simulink model "IRSensor"  (R2023b)
settings: Solver=FixedStepDiscrete  StartTime=0.0  StopTime=10.0  FixedStep=0.01  RelTol=1e-3
settings Model: Creator=LENOVO-MCC  LastModifiedBy=LENOVO-MCC
settings OptimizationCC: DefaultParameterBehavior=Inlined  EnhancedBackFolding=on  PassReuseOutputArgsAs=Individual arguments  ZeroExternalMemoryAtStartup=off  ZeroInternalMemoryAtStartup=off  OptimizeBlockOrder=speed  DifferentSizesBufferReuse=on  OptimizationCustomize=off  EfficientTunableParamExpr=on
settings DebuggingCC: ParameterTunabilityLossMsg=error
settings SFSimCC: MATLABDynamicMemAlloc=off
settings RTWCC: Description=Embedded Coder  SystemTargetFile=ert.tlc  GenCodeOnly=on  TemplateMakefile=ert_default_tmf  GenerateReport=on  LaunchReport=on  GenerateCodeMetricsReport=on
settings CodeAppCC: ForceParamTrailComments=on  IgnoreCustomStorageClasses=off  OperatorAnnotations=on  SimulinkDataObjDesc=on  SFDataObjDesc=on  InsertBlockDesc=on
settings ERTTargetCC: TargetLangStandard=C99 (ISO)  GenerateSampleERTMain=on  InlinedParameterPlacement=NonHierarchical  ERTCustomFileTemplate=example_file_process.tlc

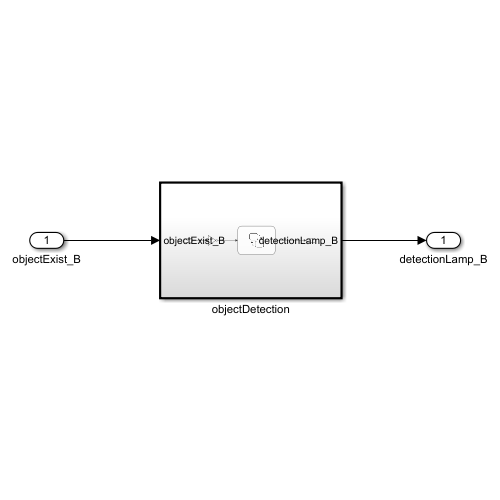
[thumbnail: Simulink's stored preview of the top-level diagram]
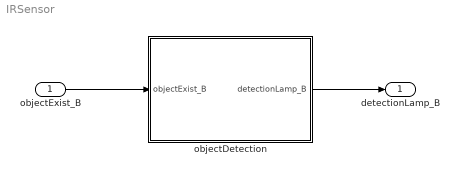
== system IRSensor ==
  objectExist_B : Inport  OutDataTypeStr=boolean
  objectDetection : Subsystem  TreatAsAtomicUnit=on
      settings: RTWFcnNameOpts=Use subsystem name  RTWFileNameOpts=Use subsystem name
  detectionLamp_B : Outport  OutDataTypeStr=boolean
  wires:
  objectExist_B/1 -> objectDetection/1(objectExist_B)
  objectDetection/1(detectionLamp_B) -> detectionLamp_B/1

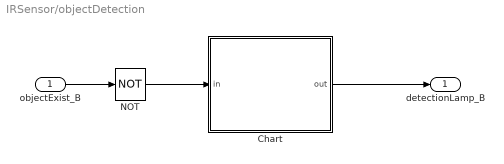
== system IRSensor/objectDetection ==
  objectExist_B : Inport  OutDataTypeStr=boolean
  Chart : Stateflow chart  TreatAsAtomicUnit=on
  NOT : Logic  Operator=NOT  IconShape=distinctive  AllPortsSameDT=off  OutDataTypeStr=boolean
  detectionLamp_B : Outport  OutDataTypeStr=boolean
  wires:
  objectExist_B/1 -> NOT/1
  NOT/1 -> Chart/1(in)
  Chart/1(out) -> detectionLamp_B/1

== stateflow chart IRSensor/objectDetection/Chart ==
  state init
    en:
    out = false;
  state hold
    en:
    counter = 0;
    du:
    counter = counter + 1;
    out = true;
  (default) -> init
  init -> hold : [in == true]
  hold -> init : [counter >= 20]
  data: in input boolean; out output boolean; counter local uint8
